simulink subsystem "Gyroscope_SubSystem"  (R2020b)
settings: Solver=VariableStepAuto  StartTime=0.0  StopTime=10.0  RelTol=1e-3
values from neighbouring files (symbols this model uses):
  Ts = 1e-2    (= 0.01)    [balrob_params.m]
settings Model: Creator=umberto  LastModifiedBy=umberto

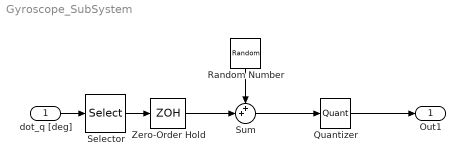
== system Gyroscope_SubSystem ==
  dot_q [deg] : Inport
  Quantizer : Quantizer  QuantizationInterval=sens.mpu.gyro.LSB2degs
  Random Number : RandomNumber  Variance=sens.mpu.gyro.noisevar  SampleTime=Ts
  Selector : Selector  InputPortWidth=2  IndexOptions=Index vector (dialog)  Indices=[2]  OutputSizes=1
  Sum : Sum  Inputs=++|
  Zero-Order Hold : ZeroOrderHold  SampleTime=Ts
  Out1 : Outport
  wires:
  dot_q [deg]/1 -> Selector/1
  Quantizer/1 -> Out1/1
  Selector/1 -> Zero-Order Hold/1
  Zero-Order Hold/1 -> Sum/2
  Sum/1 -> Quantizer/1
  Random Number/1 -> Sum/1
